simulink model "thetaupdate_new"  (R2018b)
settings: Solver=VariableStepAuto  StartTime=0.0  StopTime=10.0  RelTol=1e-3
undefined symbols (not defined in the file or in its folder): g, s, theta, Torque
settings Model: Creator=mishray  LastModifiedBy=mishray

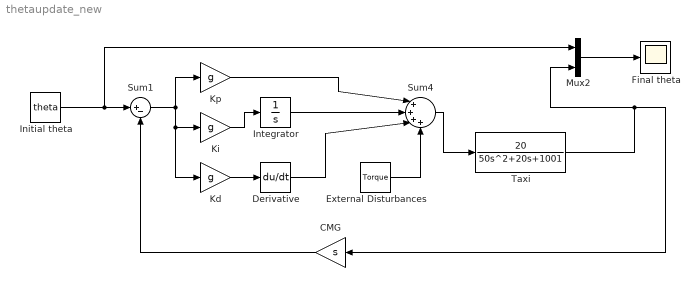
== system thetaupdate_new ==
  CMG : Gain  Gain=s
  Derivative : Derivative
  External Disturbances : Constant  Value=Torque
  Final theta : Scope
  Initial theta : Constant  Value=theta
  Integrator : Integrator
  Kd : Gain  Gain=g
  Ki : Gain  Gain=g
  Kp : Gain  Gain=g
  Mux2 : Mux  Inputs=2
  Sum1 : Sum  Inputs=|+-
  Sum4 : Sum  Inputs=|++++
  Taxi : TransferFcn  Numerator=[20]  Denominator=[50 20 1001]
  wires:
  CMG/1 -> Sum1/2
  Integrator/1 -> Sum4/2
  Ki/1 -> Integrator/1
  External Disturbances/1 -> Sum4/4
  Derivative/1 -> Sum4/3
  Sum4/1 -> Taxi/1
  Initial theta/1 -> Mux2/1, Sum1/1
  Taxi/1 -> Mux2/2, CMG/1
  Kd/1 -> Derivative/1
  Kp/1 -> Sum4/1
  Sum1/1 -> Kd/1, Ki/1, Kp/1
  Mux2/1 -> Final theta/1
